simulink model "bpswnymf"  (Simulink 5.0)
settings: Solver=ode45  StartTime=0.0  StopTime=999999  MaxStep=.0010  MinStep=0.000001  RelTol=1e-6  AbsTol=1e-6
values from neighbouring files (symbols this model uses):
  den = real(poly(p(v:v+1)))    [bwthui.m]    (also in rcosfltk.m = 3)
  num = real(poly(z(index)))    [bwthui.m]    (also in rcosfltk.m = 0.5)
undefined symbols (not defined in the file or in its folder): eyediasi, eyesampl
libraries: librnew x2
CloseFcn:
  | closemodcross
settings Model: Creator=gerhard  LastModifiedBy=bauch  ExtModeAutoUpdateStatusClock=off  SaveTime=off  SaveOutput=off  BlockReductionOpt=off  BooleanDataType=off

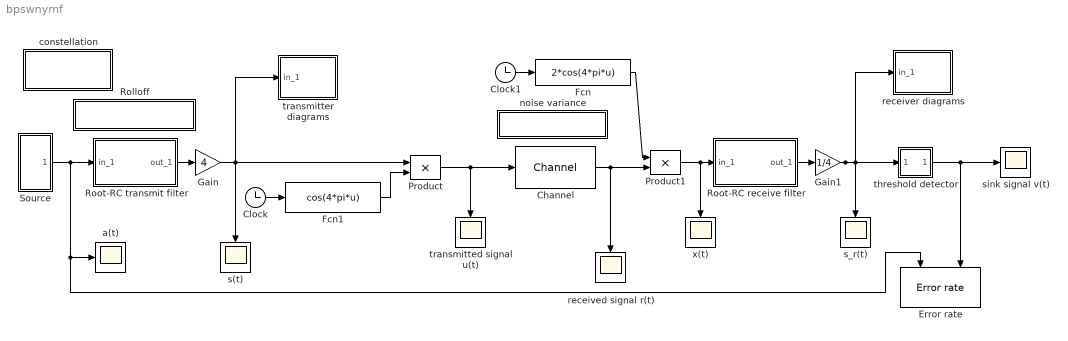
== system bpswnymf ==
  Channel : librnew/Channel  m=0  variance=0.001  s=12345
  Clock : Clock
      settings: Decimation=10
  Clock1 : Clock
      settings: Decimation=10
  Error rate : librnew/Error rate  Orientation=down  MaskParam1=1  MaskParam2=10  MaskParam3=12  MaskParam4=1
  Fcn : Fcn  Expr=2*cos(4*pi*u)
  Fcn1 : Fcn  Expr=cos(4*pi*u)
  Gain : Gain  Gain=4  SaturateOnIntegerOverflow=on
  Gain1 : Gain  Gain=1/4  SaturateOnIntegerOverflow=on
  Product : Product  SaturateOnIntegerOverflow=on  InputSameDT=on
  Product1 : Product  SaturateOnIntegerOverflow=on  InputSameDT=on
  Rolloff : Subsystem
      settings: OpenFcn=setrobin
      mask Type: rolloff
      mask Display: disp('Rolloff-Factor')
  Root-RC receive filter : Subsystem  mask(R-C filter){@1=1, @2=.05, @3=0.5, @4=6, @5='FIR/Sqrt', @6=0}
      mask prompts: @1 "Symbol interval (sec):"; @2 "Computation sampling time (sec):"; @3 "Filter rolloff factor:"; @4 "Delay step (integer to multiply symbol interval):"; @5 "Filter type (FIR or IIR) / (Normal or Sqrt):"; @6 "With or without sinc filter (1 or 0, suggest 1):"
      mask help: Design a raised cosine filter and use it to filter the input signal.
      mask init:
      | td=@1;if length(td)>1,off=td(2);td=td(1);else,off=0;end;ts=@2;R=@3;delay=@4;fil=@5;[num,den]=rcosine(1/td(1),1/ts(1),fil,R,delay);x=@6/2;
      mask Help: This block designs a raised cosine filter using the specified parameter. The filter is used to filter the input signal. You can optionally use the sinc filter in the filtering computation.
      mask Display: disp('R-C\nfilter')
  Root-RC transmit filter : Subsystem  mask(R-C filter){@1=1, @2=.05, @3=0.5, @4=6, @5='FIR/Sqrt', @6=1}
      mask prompts: @1 "Symbol interval (sec):"; @2 "Computation sampling time (sec):"; @3 "Filter rolloff factor:"; @4 "Delay step (integer to multiply symbol interval):"; @5 "Filter type (FIR or IIR) / (Normal or Sqrt):"; @6 "With or without sinc filter (1 or 0, suggest 1):"
      mask help: Design a raised cosine filter and use it to filter the input signal.
      mask init:
      | td=@1;if length(td)>1,off=td(2);td=td(1);else,off=0;end;ts=@2;R=@3;delay=@4;fil=@5;[num,den]=rcosine(1/td(1),1/ts(1),fil,R,delay);x=@6/2;
      mask Help: This block designs a raised cosine filter using the specified parameter. The filter is used to filter the input signal. You can optionally use the sinc filter in the filtering computation.
      mask Display: disp('R-C\nfilter')
  Source : Subsystem
  a(t) : Scope
      settings: TimeRange=25.000000  YMin=-2  YMax=2  DataFormat=Array
  constellation : Subsystem
      settings: OpenFcn=cplotpsk(2)
      mask Type: constellation
      mask Display: disp('Signal Space \n Constellation')
  noise variance : Subsystem
      settings: OpenFcn=setnoise
      mask Type: noise
      mask Display: disp('Noise variance')
  received signal r(t) : Scope
      settings: Orientation=down  TimeRange=25.000000  YMin=-2  YMax=2  DataFormat=Array
  receiver diagrams : Subsystem  mask(Diagrams){starttime=12, anzahl=40, offset=0}
      mask prompts: starttime "Plot start time:"; anzahl "Samples per time slot (2*T):"; offset "Decision offset:"
      mask help: Eye pattern, signal space trajectory and scatter plot.
      mask init:
      | [x, y] = srcsicon(10);
      mask Display: plot(0,0,100,100,x,y)
  s(t) : Scope
      settings: Orientation=down  TimeRange=25.000000  YMin=-2  YMax=2  DataFormat=Array
  s_r(t) : Scope
      settings: Orientation=down  TimeRange=25.000000  YMin=-2  YMax=2  DataFormat=Array
  sink signal v(t) : Scope
      settings: TimeRange=25.000000  YMin=-2  YMax=2  DataFormat=Array
  threshold detector : Subsystem
      mask Type: Sign
      mask Description: y = sign(x)
      mask Help: Sign Function:\n\t\t\ty = 1 if x > 0\n\t\t\ty = 0 if x = 0\n\t\t\ty = -1 if x < 0
      mask Display: plot(-50,-50,50,50,[-50,50],[0,0],[0,0],[-50,50],[-40,0],[-30,-30],[0,40],[30,30])
  transmitted signal u(t) : Scope
      settings: Orientation=down  TimeRange=25.000000  YMin=-2  YMax=2  DataFormat=Array
  transmitter diagrams : Subsystem  mask(Diagrams){starttime=6, anzahl=40, offset=0}
      mask prompts: starttime "Plot start time:"; anzahl "samples per time slot"; offset "decision offset"
      mask help: Eye pattern, signal-space trajectory and scatter plot
      mask init:
      | [x, y] = srcsicon(10);
      mask Display: plot(0,0,100,100,x,y)
  x(t) : Scope
      settings: Orientation=down  TimeRange=25.000000  YMin=-2  YMax=2  DataFormat=Array
  wires:
  Clock/1 -> Fcn1/1
  Fcn/1 -> Product1/1
  Clock1/1 -> Fcn/1
  threshold detector/1(out_1) -> sink signal v(t)/1, Error rate/2
  Fcn1/1 -> Product/2
  Product/1 -> transmitted signal u(t)/1, Channel/1
  Channel/1 -> Product1/2, received signal r(t)/1
  Source/1(out_1) -> Root-RC transmit filter/1(in_1), a(t)/1, Error rate/1
  Product1/1 -> Root-RC receive filter/1(in_1), x(t)/1
  Gain/1 -> Product/1, s(t)/1, transmitter diagrams/1(in_1)
  Root-RC transmit filter/1(out_1) -> Gain/1
  Root-RC receive filter/1(out_1) -> Gain1/1
  Gain1/1 -> threshold detector/1(in_1), s_r(t)/1, receiver diagrams/1(in_1)

== system bpswnymf/Rolloff ==

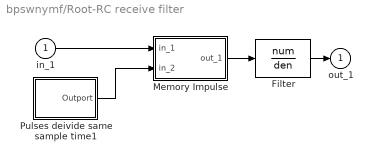
== system bpswnymf/Root-RC receive filter ==
  in_1 : Inport
  Filter : DiscreteFilter  Numerator=num  Denominator=den  SampleTime=ts
  Memory Impulse : Subsystem  mask(Impulse){@1=ts, @2=x}
      mask prompts: @1 "Holding time:"; @2 "Threshold for clock pulse:"
      mask help: 1/sinc filter:
      mask init:
      | ts=@1;thr=@2;x=thr>0;
      mask Help: When the threshold is greater than zero, this block outputs an impulse signal, which begins at the raising edge of the second input and lasts the holding time. The impulse holds a constant amplitude, which equals the amplitude of the first input at the begining of the impulse. A clock raising edge will trigger next impulse. When the threshold is less or equal to zero, this block faithfully outputs the first input.
      mask Display: disp('1/sinc')
  Pulses deivide same sample time1 : Subsystem  mask(Pulse generator){@1=td, @2=1, @3=off}
      mask prompts: @1 "Sample time (scalar, sec):"; @2 "Divider (integer vector):"; @3 "Offset (have same dimension as Divider:"
      mask help: Vector pulses with sample rate of each pulse as Sample_time ./Divider.
      mask init:
      | samp_time=@1;out_divid=@2;offset=@3;
      mask Help: This block generator a vector pulses. The output length is the same as the vector defined in "Divider". The ith element of the output has the sample time Sample_time/Divider(i). All elements in "Divider" must be integers.
      mask Display: disp('Vector\nPulse')
  out_1 : Outport
  wires:
  Filter/1 -> out_1/1
  in_1/1 -> Memory Impulse/1(in_1)
  Memory Impulse/1(out_1) -> Filter/1
  Pulses deivide same sample time1/1(Outport) -> Memory Impulse/2(in_2)

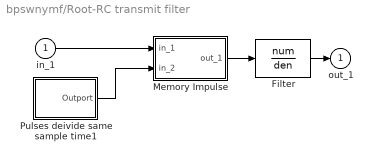
== system bpswnymf/Root-RC transmit filter ==
  in_1 : Inport
  Filter : DiscreteFilter  Numerator=num  Denominator=den  SampleTime=ts
  Memory Impulse : Subsystem  mask(Impulse){@1=ts, @2=x}
      mask prompts: @1 "Holding time:"; @2 "Threshold for clock pulse:"
      mask help: 1/sinc filter:
      mask init:
      | ts=@1;thr=@2;x=thr>0;
      mask Help: When the threshold is greater than zero, this block outputs an impulse signal, which begins at the raising edge of the second input and lasts the holding time. The impulse holds a constant amplitude, which equals the amplitude of the first input at the begining of the impulse. A clock raising edge will trigger next impulse. When the threshold is less or equal to zero, this block faithfully outputs the first input.
      mask Display: disp('1/sinc')
  Pulses deivide same sample time1 : Subsystem  mask(Pulse generator){@1=td, @2=1, @3=off}
      mask prompts: @1 "Sample time (scalar, sec):"; @2 "Divider (integer vector):"; @3 "Offset (have same dimension as Divider:"
      mask help: Vector pulses with sample rate of each pulse as Sample_time ./Divider.
      mask init:
      | samp_time=@1;out_divid=@2;offset=@3;
      mask Help: This block generator a vector pulses. The output length is the same as the vector defined in "Divider". The ith element of the output has the sample time Sample_time/Divider(i). All elements in "Divider" must be integers.
      mask Display: disp('Vector\nPulse')
  out_1 : Outport
  wires:
  Filter/1 -> out_1/1
  in_1/1 -> Memory Impulse/1(in_1)
  Memory Impulse/1(out_1) -> Filter/1
  Pulses deivide same sample time1/1(Outport) -> Memory Impulse/2(in_2)

== system bpswnymf/Source ==
  Fcn : Fcn  Expr=1-2*u
  Source : Subsystem  mask(Read from workspace){@1=randint(1000,1,2), @2=1, @3=1, @4=1}
      mask prompts: @1 "Variable (column_number=block_output_length):"; @2 "Data output sample time (sec):"; @3 "Repeat flag (1: repeat read, 0: output zeros after eof)."; @4 "Initial output:"
      mask help:
      | Read from a workspace variable at
      | sampling time point.
      mask init:
      | var=@1;td=@2;ts=td(1);if (length(td)>=2),off=td(2);else off=0;end;cyc=@3;ini=@4;[x,y]=srcsicon(7);
      mask Help: This block reads from a workspace variable at a given sample time. The column number is the block output vector length. When the simulation reaches the end of the variable (eof), the block will cyclically output from the first row of the variable or output zeros based on the repeat flag entree.
      mask Display: plot(0,0,100,100,x,y);disp('Rd wksp')
  out_1 : Outport
  wires:
  Source/1(out_1) -> Fcn/1
  Fcn/1 -> out_1/1

== system bpswnymf/constellation ==

== system bpswnymf/noise variance ==

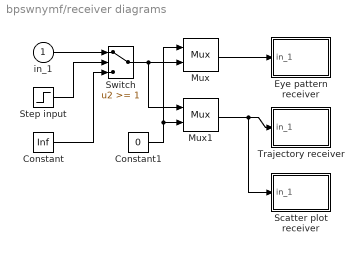
== system bpswnymf/receiver diagrams ==
  in_1 : Inport
  Constant : Constant  Value=Inf
  Constant1 : Constant  Value=0
  Eye pattern receiver : Subsystem  LoadFcn=eyesampl([],[],[],'LoadBlock')  StartFcn=eyesampl([],[],[],'Start')  StopFcn=eyesampl([],[],[],'Stop')  mask(Eye-diagram/scatter plot){@1=[2 0 1+offset], @2=[-1.5 1.5], @3=0, @4='w-/r-', @5=0, @6=2/anzahl}
      mask prompts: @1 "[Symbol interval, plot offset, decision point offset]:"; @2 "Lower and upper bound of in-coming signal (1x2 vector):"; @3 "Number of saved traces:"; @4 "Line-type for eye-pattern diagram (0 for no plot):"; @5 "Line-type for scatter plot (0 for no plot):"; @6 "Plot update sample time:"
      mask help: Produce eye-pattern diagram and/or scatter plot.
      mask init:
      | time_range=@1;boundary=@2;kept_length=@3;eye_line=@4;scatter_line=@5;two_d_line=@6;[x,y]=srcsicon(10);
      settings: CopyFcn=eyesampl([],[],[],'CopyBlock')  DeleteFcn=eyesampl([],[],[],'DeleteBlock')  NameChangeFcn=eyesampl([],[],[],'NameChange')
      mask Help: This plot opens one, or two plots by assigning the line type parameters. The scatter plot point is selected by the decision point in the first parameter entry. A decision line is drawn in the eye-pattern diagram. The plot is updated at the plot update sample time point.
      mask Display: plot(0,0,100,100,x,y);
  Mux : Mux  Inputs=2
  Mux1 : Mux  Inputs=2
  Scatter plot receiver : Subsystem  LoadFcn=eyesampl([],[],[],'LoadBlock')  StartFcn=eyesampl([],[],[],'Start')  StopFcn=eyesampl([],[],[],'Stop')  mask(Eye-diagram/scatter plot){@1=[1 .5 .999], @2=[-1.5 1.5], @3=0, @4=0, @5='b.', @6=[.5 offset]}
      mask prompts: @1 "[Symbol interval, plot offset, decision point offset]:"; @2 "Lower and upper bound of in-coming signal (1x2 vector):"; @3 "Number of saved traces:"; @4 "Line-type for eye-pattern diagram (0 for no plot):"; @5 "Line-type for scatter plot (0 for no plot):"; @6 "Plot update sample time:"
      mask help: Produce eye-pattern diagram and/or scatter plot.
      mask init:
      | time_range=@1;boundary=@2;kept_length=@3;eye_line=@4;scatter_line=@5;two_d_line=@6;[x,y]=srcsicon(10);
      settings: CopyFcn=eyesampl([],[],[],'CopyBlock')  DeleteFcn=eyesampl([],[],[],'DeleteBlock')  NameChangeFcn=eyesampl([],[],[],'NameChange')
      mask Help: This plot opens one, or two plots by assigning the line type parameters. The scatter plot point is selected by the decision point in the first parameter entry. A decision line is drawn in the eye-pattern diagram. The plot is updated at the plot update sample time point.
      mask Display: plot(0,0,100,100,x,y);
  Step input : Step  Time=starttime  SampleTime=1
  Switch : Switch  Threshold=1  SaturateOnIntegerOverflow=on  InputSameDT=on
  Trajectory receiver : Subsystem  LoadFcn=eyediasi([],[],[],'LoadBlock')  StartFcn=eyediasi([],[],[],'Start')  StopFcn=eyediasi([],[],[],'Stop')  mask(Eye-diagram/scatter plot){@1=[2 0 1], @2=[-1.5 1.5], @3=0, @4=0, @5=0, @6='g-'}
      mask prompts: @1 "Eye-pattern plot time frame:"; @2 "Lower and upper bound of in-coming signal (1x2 vector):"; @3 "Number of saved traces:"; @4 "Line-type for eye-pattern diagram (0 for no plot):"; @5 "Line-type for scatter plot (0 for no plot):"; @6 "Line-type for x-y plot (0 for no plot):"
      mask help:
      | Produce eye-pattern diagram/scatter
      | plot/x-y plot with the rising edge of the second input as the decision line.
      mask init:
      | time_range=@1;boundary=@2;kept_length=@3;eye_line=@4;scatter_line=@5;two_d_line=@6;[x,y]=srcsicon(10);[v,w]=trigicon(0,25,get_param(gcb,'orientation'),2);
      settings: CopyFcn=eyediasi([],[],[],'CopyBlock')  DeleteFcn=eyediasi([],[],[],'DeleteBlock')  NameChangeFcn=eyediasi([],[],[],'NameChange')
      mask Help: This plot opens one, two, or three plots by assigning the line type parameters. The scatter plot point is selected by the rising edge of a trigger signal. A decision line is drawn at the rising edge of the trigger signal.
      mask Display: plot(0,0,100,100,x,y,v,w);
  wires:
  Mux/1 -> Eye pattern receiver/1(in_1)
  in_1/1 -> Switch/1
  Step input/1 -> Switch/2
  Constant/1 -> Switch/3
  Mux1/1 -> Trajectory receiver/1(in_1), Scatter plot receiver/1(in_1)
  Constant1/1 -> Mux/1, Mux1/2
  Switch/1 -> Mux/2, Mux1/1

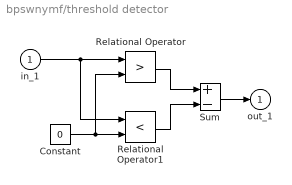
== system bpswnymf/threshold detector ==
  in_1 : Inport
  Constant : Constant  Value=0
  Relational Operator : RelationalOperator  Operator=>  InputSameDT=on
  Relational Operator1 : RelationalOperator  Operator=<  InputSameDT=on
  Sum : Sum  Inputs=+-  SaturateOnIntegerOverflow=on  InputSameDT=on
  out_1 : Outport
  wires:
  Sum/1 -> out_1/1
  Relational Operator/1 -> Sum/1
  Relational Operator1/1 -> Sum/2
  Constant/1 -> Relational Operator1/2, Relational Operator/2
  in_1/1 -> Relational Operator/1, Relational Operator1/1

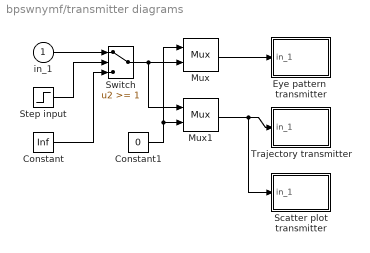
== system bpswnymf/transmitter diagrams ==
  in_1 : Inport
  Constant : Constant  Value=Inf
  Constant1 : Constant  Value=0
  Eye pattern  transmitter : Subsystem  LoadFcn=eyesampl([],[],[],'LoadBlock')  StartFcn=eyesampl([],[],[],'Start')  StopFcn=eyesampl([],[],[],'Stop')  mask(Eye-diagram/scatter plot){@1=[2 0 1+offset], @2=[-1.5 1.5], @3=0, @4='w-/r-', @5=0, @6=2/anzahl}
      mask prompts: @1 "[Symbol interval, plot offset, decision point offset]:"; @2 "Lower and upper bound of in-coming signal (1x2 vector):"; @3 "Number of saved traces:"; @4 "Line-type for eye-pattern diagram (0 for no plot):"; @5 "Line-type for scatter plot (0 for no plot):"; @6 "Plot update sample time:"
      mask help: Produce eye-pattern diagram and/or scatter plot.
      mask init:
      | time_range=@1;boundary=@2;kept_length=@3;eye_line=@4;scatter_line=@5;two_d_line=@6;[x,y]=srcsicon(10);
      settings: CopyFcn=eyesampl([],[],[],'CopyBlock')  DeleteFcn=eyesampl([],[],[],'DeleteBlock')  NameChangeFcn=eyesampl([],[],[],'NameChange')
      mask Help: This plot opens one, or two plots by assigning the line type parameters. The scatter plot point is selected by the decision point in the first parameter entry. A decision line is drawn in the eye-pattern diagram. The plot is updated at the plot update sample time point.
      mask Display: plot(0,0,100,100,x,y);
  Mux : Mux  Inputs=2
  Mux1 : Mux  Inputs=2
  Scatter plot transmitter : Subsystem  LoadFcn=eyesampl([],[],[],'LoadBlock')  StartFcn=eyesampl([],[],[],'Start')  StopFcn=eyesampl([],[],[],'Stop')  mask(Eye-diagram/scatter plot){@1=[1 .5 .999], @2=[-1.5 1.5], @3=0, @4=0, @5='b.', @6=[.5 offset]}
      mask prompts: @1 "[Symbol interval, plot offset, decision point offset]:"; @2 "Lower and upper bound of in-coming signal (1x2 vector):"; @3 "Number of saved traces:"; @4 "Line-type for eye-pattern diagram (0 for no plot):"; @5 "Line-type for scatter plot (0 for no plot):"; @6 "Plot update sample time:"
      mask help: Produce eye-pattern diagram and/or scatter plot.
      mask init:
      | time_range=@1;boundary=@2;kept_length=@3;eye_line=@4;scatter_line=@5;two_d_line=@6;[x,y]=srcsicon(10);
      settings: CopyFcn=eyesampl([],[],[],'CopyBlock')  DeleteFcn=eyesampl([],[],[],'DeleteBlock')  NameChangeFcn=eyesampl([],[],[],'NameChange')
      mask Help: This plot opens one, or two plots by assigning the line type parameters. The scatter plot point is selected by the decision point in the first parameter entry. A decision line is drawn in the eye-pattern diagram. The plot is updated at the plot update sample time point.
      mask Display: plot(0,0,100,100,x,y);
  Step input : Step  Time=starttime  SampleTime=1
  Switch : Switch  Threshold=1  SaturateOnIntegerOverflow=on  InputSameDT=on
  Trajectory transmitter : Subsystem  LoadFcn=eyediasi([],[],[],'LoadBlock')  StartFcn=eyediasi([],[],[],'Start')  StopFcn=eyediasi([],[],[],'Stop')  mask(Eye-diagram/scatter plot){@1=[2 0 1], @2=[-1.5 1.5], @3=0, @4=0, @5=0, @6='g-'}
      mask prompts: @1 "Eye-pattern plot time frame:"; @2 "Lower and upper bound of in-coming signal (1x2 vector):"; @3 "Number of saved traces:"; @4 "Line-type for eye-pattern diagram (0 for no plot):"; @5 "Line-type for scatter plot (0 for no plot):"; @6 "Line-type for x-y plot (0 for no plot):"
      mask help:
      | Produce eye-pattern diagram/scatter
      | plot/x-y plot with the rising edge of the second input as the decision line.
      mask init:
      | time_range=@1;boundary=@2;kept_length=@3;eye_line=@4;scatter_line=@5;two_d_line=@6;[x,y]=srcsicon(10);[v,w]=trigicon(0,25,get_param(gcb,'orientation'),2);
      settings: CopyFcn=eyediasi([],[],[],'CopyBlock')  DeleteFcn=eyediasi([],[],[],'DeleteBlock')  NameChangeFcn=eyediasi([],[],[],'NameChange')
      mask Help: This plot opens one, two, or three plots by assigning the line type parameters. The scatter plot point is selected by the rising edge of a trigger signal. A decision line is drawn at the rising edge of the trigger signal.
      mask Display: plot(0,0,100,100,x,y,v,w);
  wires:
  Switch/1 -> Mux/2, Mux1/1
  Constant1/1 -> Mux/1, Mux1/2
  Mux1/1 -> Trajectory transmitter/1(in_1), Scatter plot transmitter/1(in_1)
  Constant/1 -> Switch/3
  Step input/1 -> Switch/2
  in_1/1 -> Switch/1
  Mux/1 -> Eye pattern  transmitter/1(in_1)

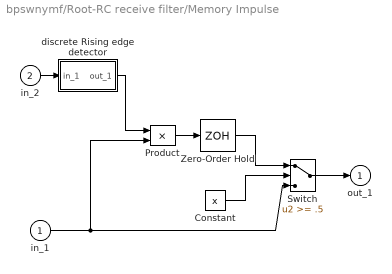
== system bpswnymf/Root-RC receive filter/Memory Impulse ==
  in_1 : Inport
  in_2 : Inport  Port=2
  Constant : Constant  Value=x
  Product : Product  SaturateOnIntegerOverflow=on  InputSameDT=on
  Switch : Switch  Threshold=.5  SaturateOnIntegerOverflow=on  InputSameDT=on
  Zero-Order Hold : ZeroOrderHold  SampleTime=ts
  discrete Rising edge detector : Subsystem  mask(Edge Detection){@1=thr, @2=ts}
      mask prompts: @1 "Threshold:"; @2 "Sampling time:"
      mask help: Rising edge detection:
      mask init:
      | thld=@1;ts=@2;
      mask Help: When the input signal rising edge passed the given shreshold, this block outputs one, otherwise outputs zero.
      mask Display: disp('Edge\nDetector')
  out_1 : Outport
  wires:
  in_2/1 -> discrete Rising edge detector/1(in_1)
  discrete Rising edge detector/1(out_1) -> Product/1
  Constant/1 -> Switch/2
  Switch/1 -> out_1/1
  in_1/1 -> Switch/3, Product/2
  Product/1 -> Zero-Order Hold/1
  Zero-Order Hold/1 -> Switch/1

== system bpswnymf/Root-RC receive filter/Pulses deivide same sample time1 ==
  S-function1 : S-Function  FunctionName=homopuls  Parameters=samp_time, out_divid, offset
  Outport : Outport
  wires:
  S-function1/1 -> Outport/1

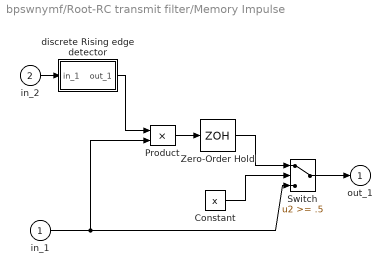
== system bpswnymf/Root-RC transmit filter/Memory Impulse ==
  in_1 : Inport
  in_2 : Inport  Port=2
  Constant : Constant  Value=x
  Product : Product  SaturateOnIntegerOverflow=on  InputSameDT=on
  Switch : Switch  Threshold=.5  SaturateOnIntegerOverflow=on  InputSameDT=on
  Zero-Order Hold : ZeroOrderHold  SampleTime=ts
  discrete Rising edge detector : Subsystem  mask(Edge Detection){@1=thr, @2=ts}
      mask prompts: @1 "Threshold:"; @2 "Sampling time:"
      mask help: Rising edge detection:
      mask init:
      | thld=@1;ts=@2;
      mask Help: When the input signal rising edge passed the given shreshold, this block outputs one, otherwise outputs zero.
      mask Display: disp('Edge\nDetector')
  out_1 : Outport
  wires:
  in_2/1 -> discrete Rising edge detector/1(in_1)
  discrete Rising edge detector/1(out_1) -> Product/1
  Constant/1 -> Switch/2
  Switch/1 -> out_1/1
  in_1/1 -> Switch/3, Product/2
  Product/1 -> Zero-Order Hold/1
  Zero-Order Hold/1 -> Switch/1

== system bpswnymf/Root-RC transmit filter/Pulses deivide same sample time1 ==
  S-function1 : S-Function  FunctionName=homopuls  Parameters=samp_time, out_divid, offset
  Outport : Outport
  wires:
  S-function1/1 -> Outport/1

== system bpswnymf/Source/Source ==
  Message source : S-Function  FunctionName=trigwksp  Parameters=var,thd,cyclFlag,ini  mask(Read from workspace){@1=var, @2=.1, @3=cyc, @4=ini}
      mask prompts: @1 "Read the variable:"; @2 "Threshold for the input pulse:"; @3 "Cyclic read variable (1) or amend zeros (0)."; @4 "Output before first trigger:"
      mask help: The raising edge of input pulse trigger the block output the next row from the workspace variable.
      mask init:
      | var=@1;thd=@2;cyclFlag=@3;ini=@4;
      mask Help: This block reads the data from a workspace variable. The output is refreshed at the raising edge of the input pulse.
      mask Display: disp('Triggered\nread')
  Pulses deivide same sample time1 : Subsystem  mask(Pulse generator){@1=ts, @2=1, @3=off}
      mask prompts: @1 "Sample time (scalar, sec):"; @2 "Divider (integer vector):"; @3 "Offset (have same dimension as Divider:"
      mask help: Vector pulses with sample rate of each pulse as Sample_time ./Divider.
      mask init:
      | samp_time=@1;out_divid=@2;offset=@3;
      mask Help: This block generator a vector pulses. The output length is the same as the vector defined in "Divider". The ith element of the output has the sample time Sample_time/Divider(i). All elements in "Divider" must be integers.
      mask Display: disp('Vector\nPulse')
  out_1 : Outport
  wires:
  Message source/1 -> out_1/1
  Pulses deivide same sample time1/1(Outport) -> Message source/1

== system bpswnymf/receiver diagrams/Eye pattern receiver ==
  in_1 : Inport
  Plot1 : S-Function  FunctionName=eyesampl  Parameters=time_range, boundary, kept_length, eye_line, scatter_line, two_d_line
  wires:
  in_1/1 -> Plot1/1

== system bpswnymf/receiver diagrams/Scatter plot receiver ==
  in_1 : Inport
  Plot1 : S-Function  FunctionName=eyesampl  Parameters=time_range, boundary, kept_length, eye_line, scatter_line, two_d_line
  wires:
  in_1/1 -> Plot1/1

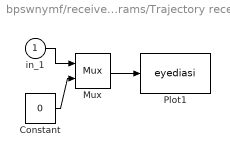
== system bpswnymf/receiver diagrams/Trajectory receiver ==
  in_1 : Inport
  Constant : Constant  Value=0
  Mux : Mux  Inputs=2
  Plot1 : S-Function  FunctionName=eyediasi  Parameters=time_range, boundary, kept_length, eye_line, scatter_line, two_d_line
  wires:
  Mux/1 -> Plot1/1
  Constant/1 -> Mux/2
  in_1/1 -> Mux/1

== system bpswnymf/transmitter diagrams/Eye pattern  transmitter ==
  in_1 : Inport
  Plot1 : S-Function  FunctionName=eyesampl  Parameters=time_range, boundary, kept_length, eye_line, scatter_line, two_d_line
  wires:
  in_1/1 -> Plot1/1

== system bpswnymf/transmitter diagrams/Scatter plot transmitter ==
  in_1 : Inport
  Plot1 : S-Function  FunctionName=eyesampl  Parameters=time_range, boundary, kept_length, eye_line, scatter_line, two_d_line
  wires:
  in_1/1 -> Plot1/1

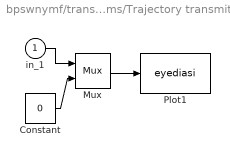
== system bpswnymf/transmitter diagrams/Trajectory transmitter ==
  in_1 : Inport
  Constant : Constant  Value=0
  Mux : Mux  Inputs=2
  Plot1 : S-Function  FunctionName=eyediasi  Parameters=time_range, boundary, kept_length, eye_line, scatter_line, two_d_line
  wires:
  in_1/1 -> Mux/1
  Constant/1 -> Mux/2
  Mux/1 -> Plot1/1

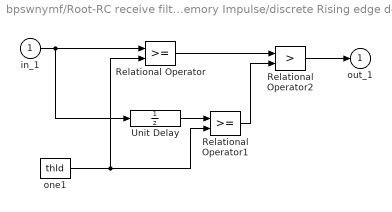
== system bpswnymf/Root-RC receive filter/Memory Impulse/discrete Rising edge detector ==
  in_1 : Inport
  Relational Operator : RelationalOperator  InputSameDT=on
  Relational Operator1 : RelationalOperator  InputSameDT=on
  Relational Operator2 : RelationalOperator  Operator=>  InputSameDT=on
  Unit Delay : UnitDelay  SampleTime=ts
  one1 : Constant  Value=thld
  out_1 : Outport
  wires:
  in_1/1 -> Relational Operator/1, Unit Delay/1
  Unit Delay/1 -> Relational Operator1/1
  one1/1 -> Relational Operator/2, Relational Operator1/2
  Relational Operator/1 -> Relational Operator2/1
  Relational Operator1/1 -> Relational Operator2/2
  Relational Operator2/1 -> out_1/1

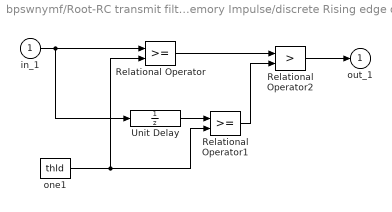
== system bpswnymf/Root-RC transmit filter/Memory Impulse/discrete Rising edge detector ==
  in_1 : Inport
  Relational Operator : RelationalOperator  InputSameDT=on
  Relational Operator1 : RelationalOperator  InputSameDT=on
  Relational Operator2 : RelationalOperator  Operator=>  InputSameDT=on
  Unit Delay : UnitDelay  SampleTime=ts
  one1 : Constant  Value=thld
  out_1 : Outport
  wires:
  in_1/1 -> Relational Operator/1, Unit Delay/1
  Unit Delay/1 -> Relational Operator1/1
  one1/1 -> Relational Operator/2, Relational Operator1/2
  Relational Operator/1 -> Relational Operator2/1
  Relational Operator1/1 -> Relational Operator2/2
  Relational Operator2/1 -> out_1/1

== system bpswnymf/Source/Source/Pulses deivide same sample time1 ==
  S-function1 : S-Function  FunctionName=homopuls  Parameters=samp_time, out_divid, offset
  Outport : Outport
  wires:
  S-function1/1 -> Outport/1
